simulink model "MultilayerProcessControlSim"  (R2023b)
settings: Solver=ode4  StartTime=0.0  StopTime=10  RelTol=1e-3
undefined symbols (not defined in the file): DiscIntNeverNeededParam
libraries: dspstat3 x22, slpidlib x14
(part 3 of 3)

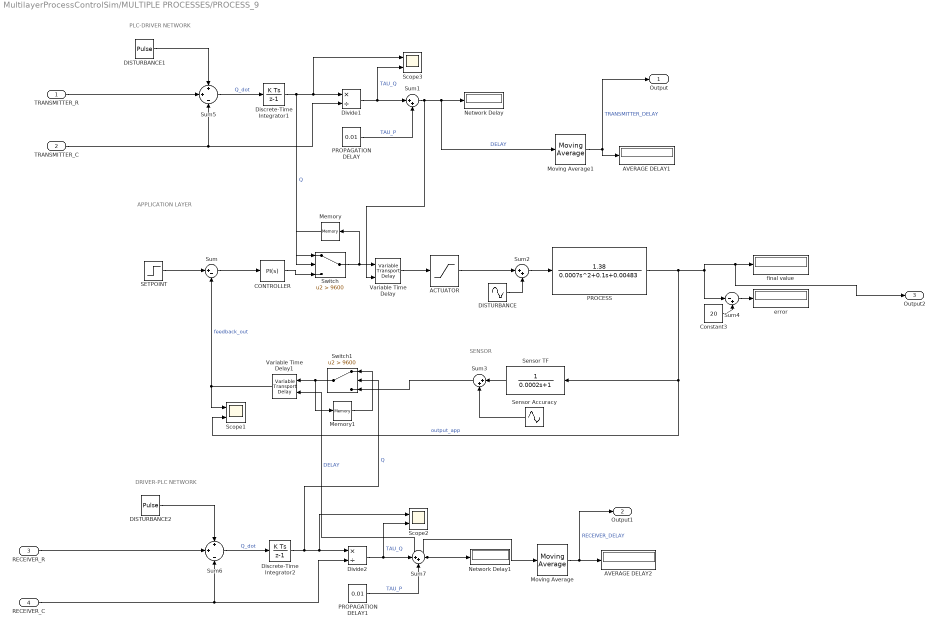
== system MultilayerProcessControlSim/MULTIPLE PROCESSES/PROCESS_9 ==
  note: SENSOR
  note: APPLICATION LAYER
  note: PLC-DRIVER NETWORK
  note: DRIVER-PLC NETWORK
  TRANSMITTER_R : Inport
  TRANSMITTER_C : Inport  Port=2
  RECEIVER_R : Inport  Port=3
  RECEIVER_C : Inport  Port=4
  ACTUATOR : Saturate  UpperLimit=150  LowerLimit=-150
  AVERAGE DELAY1 : Display
  AVERAGE DELAY2 : Display
  CONTROLLER : slpidlib/PID Controller  Controller=PI  Form=Parallel  TimeDomain=Continuous-time  UseExternalTs=off  SampleTime=-1  IntegratorMethod=Forward Euler  FilterMethod=Forward Euler  ControllerParametersSource=internal  P=1  I=3.6  UseKiTs=off  D=0  N=100  UseFilter=on  TunerSelectOption=Transfer Function Based (PID Tuner App)  InitialConditionSource=internal  InitialConditionForIntegrator=0  InitialConditionForFilter=0  DifferentiatorICPrevScaledInput=0  ExternalReset=none  TrackingMode=off  Kt=1  LimitOutput=off  SatLimitsSource=internal  UpperSaturationLimit=inf  LowerSaturationLimit=-inf  LinearizeAsGain=on  AntiWindupMode=none  Kb=1  LimitIntegrator=off  UpperIntegratorSaturationLimit=inf  LowerIntegratorSaturationLimit=-inf  POutMin=[]  POutMax=[]  IOutMin=[]  IOutMax=[]  DOutMin=[]  DOutMax=[]  NOutMin=[]  NOutMax=[]  SumOutMin=[]  SumOutMax=[]  SaturationOutMin=[]  SaturationOutMax=[]  PParamMin=[]  PParamMax=[]  IParamMin=[]  IParamMax=[]  DParamMin=[]  DParamMax=[]  NParamMin=[]  NParamMax=[]  KbParamMin=[]  KbParamMax=[]  KtParamMin=[]  KtParamMax=[]  KbOutMin=[]  KbOutMax=[]  KtOutMin=[]  KtOutMax=[]  IntegratorOutMin=[]  IntegratorOutMax=[]  FilterOutMin=[]  FilterOutMax=[]  SumI1OutMin=[]  SumI1OutMax=[]  SumI2OutMin=[]  SumI2OutMax=[]  SumI3OutMin=[]  SumI3OutMax=[]  SumI4OutMin=[]  SumI4OutMax=[]  SumDOutMin=[]  SumDOutMax=[]  DifferentiatorOutMin=[]  DifferentiatorOutMax=[]  FilterDiffOutCoefMin=[]  FilterDiffOutCoefMax=[]  ReciprocalOutMin=[]  ReciprocalOutMax=[]  SumDenOutMin=[]  SumDenOutMax=[]  SumNumOutMin=[]  SumNumOutMax=[]  DivideOutMin=[]  DivideOutMax=[]  UdiffTsProdOutMin=[]  UdiffTsProdOutMax=[]  NTsProdOutMin=[]  NTsProdOutMax=[]  UintegralTsProdOutMin=[]  UintegralTsProdOutMax=[]  UngainTsProdOutMin=[]  UngainTsProdOutMax=[]  ClampingZeroOutDataTypeStr=Inherit: Inherit via back propagation  ClampingZeroOutMin=[]  ClampingZeroOutMax=[]  FilterDenConstantOutDataTypeStr=Inherit: Inherit via back propagation  FilterDenConstantOutMin=[]  FilterDenConstantOutMax=[]  PCopyOutDataTypeStr=Inherit: Inherit via back propagation  PCopyOutMin=[]  PCopyOutMax=[]  NCopyOutDataTypeStr=Inherit: Inherit via back propagation  NCopyOutMin=[]  NCopyOutMax=[]  IntegratorContinuousStateAttributes=''  IntegratorStateMustResolveToSignalObject=off  IntegratorRTWStateStorageClass=Auto  FilterContinuousStateAttributes=''  FilterStateMustResolveToSignalObject=off  FilterRTWStateStorageClass=Auto  ParallelPVariant=InternalParameters  IdealPVariant=Disabled  IVariant=InternalParameters  DVariant=Disabled  IntegratorVariant=Continuous  SatVariant=Disabled  AWVariant=Passthrough  PCopyVariant=Disabled  TRVariant=Disabled  FdbkBlocksVariant=Forward  IdealPFdbkVariant=Disabled  SatFdbkVariant=Disabled  DerivativeFilterVariant=Disabled  NVariant=Disabled  NCopyVariant=Disabled_SignalSpec  FilterICVariant=Disabled  IntegratorICVariant=InternalICs  ExternalResetVariant=Disabled  TRSumVariant=Passthrough  SumFdbkVariant=Disabled  SumVariant=Sum_PI  TsampFilterVariant=InternalTs  TsampNgainVariant=Passthrough  TsampIntegralVariant=Disabled_SignalSpec  ExternalSaturationOutDataTypeStr=Inherit: Same as second input
  Constant3 : Constant  Value=20
  DISTURBANCE : Sin  Amplitude=0.1  Bias=0.05  Frequency=50  SampleTime=0
  DISTURBANCE1 : DiscretePulseGenerator  PulseType=Time based  Amplitude=8  Period=0.001  PulseWidth=50
  DISTURBANCE2 : DiscretePulseGenerator  PulseType=Time based  Amplitude=24  Period=0.001  PulseWidth=50
  Discrete-Time Integrator1 : DiscreteIntegrator  SampleTime=-1  LimitOutput=on  UpperSaturationLimit=9600  LowerSaturationLimit=0  ICPrevOutput=DiscIntNeverNeededParam  ICPrevScaledInput=DiscIntNeverNeededParam
  Discrete-Time Integrator2 : DiscreteIntegrator  SampleTime=-1  LimitOutput=on  UpperSaturationLimit=9600  LowerSaturationLimit=0  ICPrevOutput=DiscIntNeverNeededParam  ICPrevScaledInput=DiscIntNeverNeededParam
  Divide1 : Product  Inputs=*/
  Divide2 : Product  Inputs=*/
  Memory : Memory
  Memory1 : Memory
  Moving Average : dspstat3/Moving Average  Method=Sliding window  ForgettingFactorPort=off  SpecifyWindowLength=on  WindowLength=4  OverlapLength=3  AllowArbitraryInputLength=off  ForgettingFactor=0.9  SimulateUsing=Code generation
  Moving Average1 : dspstat3/Moving Average  Method=Sliding window  ForgettingFactorPort=off  SpecifyWindowLength=on  WindowLength=4  OverlapLength=3  AllowArbitraryInputLength=off  ForgettingFactor=0.9  SimulateUsing=Code generation
  Network Delay : Display
  Network Delay1 : Display
  PROCESS : TransferFcn  Numerator=[1.38]  Denominator=[0.0007 0.1 0.00483]
  PROPAGATION DELAY : Constant  Value=0.01
  PROPAGATION DELAY1 : Constant  Value=0.01
  SETPOINT : Step  After=20  SampleTime=0
  Scope1 : Scope  NumInputPorts=2
  Scope2 : Scope  NumInputPorts=2
  Scope3 : Scope  NumInputPorts=2
  Sensor Accuracy : Sin  Amplitude=0.01  Frequency=50  SampleTime=0
  Sensor TF : TransferFcn  Denominator=[0.0002 1]
  Sum : Sum  Inputs=|+-
  Sum{1..3,7} (4 alike) : Sum  Inputs=|++
  Sum4 : Sum  Inputs=|-+
  Sum5 : Sum  Inputs=+|+|-
  Sum6 : Sum  Inputs=+|+|-
  Switch : Switch  Criteria=u2 > Threshold  Threshold=9600  SaturateOnIntegerOverflow=off  InputSameDT=off
  Switch1 : Switch  Criteria=u2 > Threshold  Threshold=9600  SaturateOnIntegerOverflow=off  InputSameDT=off
  Variable Time Delay : VariableTransportDelay  MaximumDelay=10
  Variable Time Delay1 : VariableTransportDelay  MaximumDelay=10
  error : Display
  final value : Display
  Output : Outport
  Output1 : Outport  Port=2
  Output2 : Outport  Port=3
  wires:
  Sum/1 -> CONTROLLER/1
  DISTURBANCE/1 -> Sum2/2
  Constant3/1 -> Sum4/2
  Sum4/1 -> error/1
  Variable Time Delay/1 -> ACTUATOR/1
  PROPAGATION DELAY/1 -> Sum1/2  "TAU_P"
  Sensor TF/1 -> Sum3/1
  Sum2/1 -> PROCESS/1
  Sum5/1 -> Discrete-Time Integrator1/1  "Q_dot"
  PROPAGATION DELAY1/1 -> Sum7/2  "TAU_P"
  PROCESS/1 -> Scope1/2, Sensor TF/1, Sum4/1, final value/1, Output2/1  "output_app"
  Sum6/1 -> Discrete-Time Integrator2/1  "Q_dot"
  Sensor Accuracy/1 -> Sum3/2
  Divide1/1 -> Sum1/1, Scope3/2  "TAU_Q"
  Moving Average/1 -> AVERAGE DELAY2/1, Output1/1  "RECEIVER_DELAY"
  Divide2/1 -> Scope2/2, Sum7/1  "TAU_Q"
  Discrete-Time Integrator1/1 -> Switch/2, Divide1/1, Scope3/1  "Q"
  Variable Time Delay1/1 -> Scope1/1, Sum/2  "feedback_out"
  DISTURBANCE2/1 -> Sum6/1
  Switch1/1 -> Variable Time Delay1/1, Memory1/1
  Discrete-Time Integrator2/1 -> Divide2/1, Scope2/1, Switch1/2  "Q"
  Sum7/1 -> Network Delay1/1, Moving Average/1, Variable Time Delay1/2  "DELAY"
  SETPOINT/1 -> Sum/1
  RECEIVER_R/1 -> Sum6/2
  ACTUATOR/1 -> Sum2/1
  TRANSMITTER_R/1 -> Sum5/2
  Switch/1 -> Variable Time Delay/1, Memory/1
  Memory/1 -> Switch/1
  Memory1/1 -> Switch1/1
  Moving Average1/1 -> AVERAGE DELAY1/1, Output/1  "TRANSMITTER_DELAY"
  Sum3/1 -> Switch1/3
  CONTROLLER/1 -> Switch/3
  TRANSMITTER_C/1 -> Sum5/3, Divide1/2
  Sum1/1 -> Variable Time Delay/2, Network Delay/1, Moving Average1/1  "DELAY"
  DISTURBANCE1/1 -> Sum5/1
  RECEIVER_C/1 -> Divide2/2, Sum6/3

== system MultilayerProcessControlSim/ONE PROCESS/DRIVER-PLC NETWORK ==
  BUFFER1 : Constant  Value=120
  DISTURBANCE2 : DiscretePulseGenerator  PulseType=Time based  Amplitude=48  Period=1  PulseWidth=50
  Discrete-Time Integrator2 : DiscreteIntegrator  SampleTime=-1  LimitOutput=on  UpperSaturationLimit=9600  LowerSaturationLimit=0  ICPrevOutput=DiscIntNeverNeededParam  ICPrevScaledInput=DiscIntNeverNeededParam
  Divide2 : Product  Inputs=*/
  INPUT RATE1 : Constant  Value=96
  Network Delay1 : Display
  PROPAGATION DELAY1 : Constant  Value=0.01
  Scope2 : Scope  NumInputPorts=2
  Sum6 : Sum  Inputs=+|+|-
  Sum7 : Sum  Inputs=|++
  Q : Outport
  DELAY1 : Outport  Port=2
  wires:
  INPUT RATE1/1 -> Sum6/2
  PROPAGATION DELAY1/1 -> Sum7/2  "TAU_P"
  Discrete-Time Integrator2/1 -> Q/1, Scope2/1, Divide2/1  "Q"
  Divide2/1 -> Sum7/1, Scope2/2  "TAU_Q"
  Sum6/1 -> Discrete-Time Integrator2/1  "Q_dot"
  DISTURBANCE2/1 -> Sum6/1
  BUFFER1/1 -> Sum6/3, Divide2/2
  Sum7/1 -> Network Delay1/1, DELAY1/1  "DELAY"

== system MultilayerProcessControlSim/ONE PROCESS/PLC-DRIVER NETWORK ==
  BUFFER : Constant  Value=96
  DISTURBANCE1 : DiscretePulseGenerator  PulseType=Time based  Amplitude=48  Period=1  PulseWidth=50
  Discrete-Time Integrator1 : DiscreteIntegrator  SampleTime=-1  LimitOutput=on  UpperSaturationLimit=9600  LowerSaturationLimit=0  ICPrevOutput=DiscIntNeverNeededParam  ICPrevScaledInput=DiscIntNeverNeededParam
  Divide1 : Product  Inputs=*/
  INPUT RATE : Constant  Value=72
  Network Delay : Display
  PROPAGATION DELAY : Constant  Value=0.01
  Scope3 : Scope  NumInputPorts=2
  Sum1 : Sum  Inputs=|++
  Sum5 : Sum  Inputs=+|+|-
  DELAY1 : Outport
  Q : Outport  Port=2
  wires:
  Discrete-Time Integrator1/1 -> Divide1/1, Q/1, Scope3/1  "Q"
  DISTURBANCE1/1 -> Sum5/1
  INPUT RATE/1 -> Sum5/2
  BUFFER/1 -> Divide1/2, Sum5/3
  Divide1/1 -> Scope3/2, Sum1/1  "TAU_Q"
  PROPAGATION DELAY/1 -> Sum1/2  "TAU_P"
  Sum5/1 -> Discrete-Time Integrator1/1  "Q_dot"
  Sum1/1 -> Network Delay/1, DELAY1/1  "DELAY"
